simulink model "volo_agcdc_pipelined"  (R2012b)
settings: Solver=ode45  StartTime=0.0  StopTime=1000  RelTol=1e-3
PreLoadFcn:
  | volo_agcdc_init
InitFcn:
  | volo_agcdc_init
StartFcn:
  | volo_agcdc_init
values from neighbouring files (symbols this model uses):
  agc_idleState = 0    [volo_agcdc_init.m]
  agc_numAddrBits = agc_numOutputs + agc_numStateBits    [volo_agcdc_init.m]
  regDCRemoval_AvgLength = 64    [volo_agcdc_init.m]
  regSatDet_NumSamples = 16    [volo_agcdc_init.m]
undefined symbols (not defined in the file or in its folder): gcbh, xlBlockLoadCallback, xlGetNormalizedPeriod
libraries: xbsIndex_r4 x681, xbsEDKLib_r4 x1
(part 1 of 7)
settings Model: Creator=rng  LastModifiedBy=rng

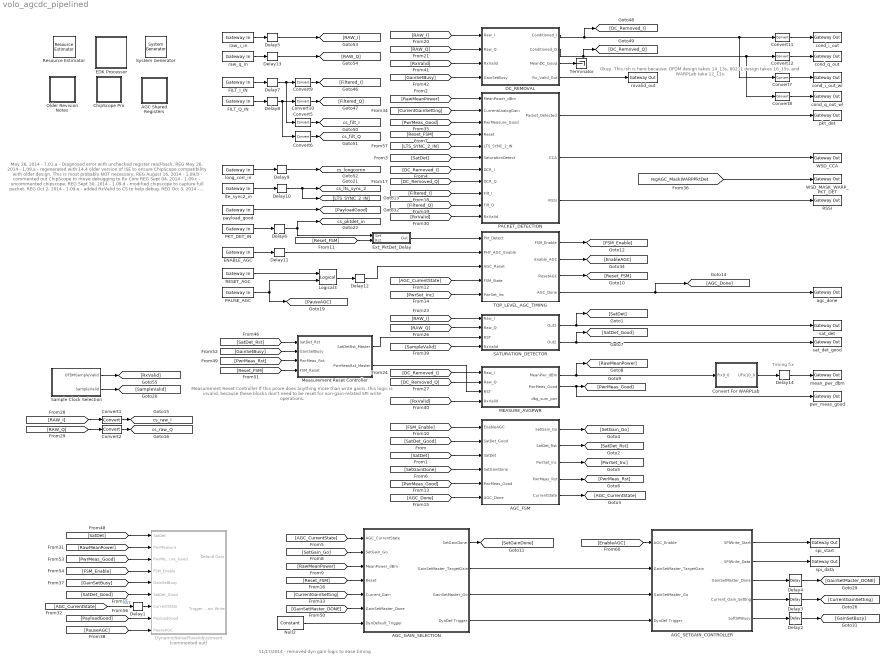
== system volo_agcdc_pipelined ==
  note: 11/17/2014 - removed dyn gain logic to ease timing
  note: Timing fix
  note: Okay. This ish is here because:
      | OFDM design takes 14_13s,
      | 80211 design takes 16_15s,
      | and WARPLab take 12_11s.
  note: May 26, 2014 - 7.01.a - Diagnosed error with unchecked register read-back. REG
      | May 26, 2014 - 1.09.a - regenerated with 14.4 older version of ISE to ensure
      | ChipScope compatibility with older design. This is most probably NOT necessary. REG
      | August 16, 2014 - 1.09.b - commented out ChipScope to move debugging to Rx Core REG
      | Sept 04, 2014 - 1.09.c - uncommented chipscope. REG
      | Sept 30, 2014 - 1.09.d - modified chipscope to capture full packet. REG
      | Oct 2, 2014 - 1.09.e - added RxValid to CS to help debug. REG
      | Oct 3, 2014 - 1.09.f - removed chipscope to wlan_phy_rx. Added RxValid output. REG
      | Nov 16, 2014 - 1.09.g - added a bit of precision to regAGC_WSD_CCAThreshold_dBm
      | MM register to make it Fix_10_0 to match comparison value. Default value now -40 dBm,
      | since the power measurement block does not current consider the external LNA in its input
      | power calculation. In later revisions, we should consider addressing this issue, but for now
      | it is more important that the RSSI and CCA value be relatively accurate and CCA thresh not
      | too low. Also re-enabled chipscope. Added CCA enable line. REG
      | Nov 17, 2014 - 1.09.h - Removed DynDefaultGain functionality to ease timing
      | requirements. REG
      | Jan 01, 2015 - 1.09.j - Added piplining on the SPI go signal, as it was needed when
      | added the 4x1 radio MUX to close timing. REG
  note: Measurement Reset Controller
      | If this pcore does anything more than write gains, this logic is invalid,
      | because these blocks don't need to be reset for non-gain-related SPI
      | write operations.
  " System Generator" : xbsIndex_r4/ System Generator  Tag=genX  xilinxfamily=virtex6  part=xc6vlx240t  speed=-2  package=ff1156  synthesis_tool=XST  clock_wrapper=Clock Enables  directory=./volo_agcdc_generated_pcores  proj_type=Project Navigator  Synth_file=XST Defaults  Impl_file=ISE Defaults  testbench=off  simulink_period=1  sysclk_period=10  dcm_input_clock_period=100  incr_netlist=off  trim_vbits=Everywhere in SubSystem  dbl_ovrd=According to Block Masks  core_generation=According to Block Masks  run_coregen=off  deprecated_control=off  eval_field=0  block_type=sysgen
      settings: block_version=10.1.3
  AGC Shared Registers : Subsystem
  AGC_FSM : Subsystem
  AGC_GAIN_SELECTION : Subsystem
  AGC_SETGAIN_CONTROLLER : Subsystem
  ChipScope Pro : Subsystem
  Convert For WARPLab : Subsystem
  Convert{1..2,5..6} (4 alike) : xbsIndex_r4/Convert  gui_display_data_type=Fixed-point  arith_type="Signed  (2's comp)"  n_bits=12  bin_pt=11  float_type=Single  exp_bits=8  fraction_bits=24  quantization="Round  (unbiased: Even Values)"  overflow=Saturate  en=off  latency=0  dbl_ovrd=off  pipeline=off  block_type=convert
  Convert{7..10} (4 alike) : xbsIndex_r4/Convert  gui_display_data_type=Fixed-point  arith_type="Signed  (2's comp)"  n_bits=12  bin_pt=11  float_type=Single  exp_bits=8  fraction_bits=24  quantization=Truncate  overflow=Wrap  en=off  latency=0  dbl_ovrd=off  pipeline=off  block_type=convert
  Convert11 : xbsIndex_r4/Convert  gui_display_data_type=Fixed-point  arith_type="Signed  (2's comp)"  n_bits=16  bin_pt=15  float_type=Single  exp_bits=8  fraction_bits=24  quantization=Truncate  overflow=Wrap  en=off  latency=0  dbl_ovrd=off  pipeline=off  block_type=convert
  Convert12 : xbsIndex_r4/Convert  gui_display_data_type=Fixed-point  arith_type="Signed  (2's comp)"  n_bits=16  bin_pt=15  float_type=Single  exp_bits=8  fraction_bits=24  quantization=Truncate  overflow=Wrap  en=off  latency=0  dbl_ovrd=off  pipeline=off  block_type=convert
  DC_REMOVAL : Subsystem
  Delay{1,5..14} (11 alike) : xbsIndex_r4/Delay  rst=off  infoeditControl=Selection of Reset will increase slice count due to use of real FFs and instead of SRLs  en=off  latency=1  dbl_ovrd=off  reg_retiming=off  block_type=delay
  Delay2 : xbsIndex_r4/Delay  rst=off  infoeditControl=Selection of Reset will increase slice count due to use of real FFs and instead of SRLs  en=off  latency=2  dbl_ovrd=off  reg_retiming=off  block_type=delay
  Delay3 : xbsIndex_r4/Delay  rst=off  infoeditControl=Selection of Reset will increase slice count due to use of real FFs and instead of SRLs  en=off  latency=2  dbl_ovrd=off  reg_retiming=off  block_type=delay
  Delay4 : xbsIndex_r4/Delay  rst=off  infoeditControl=Selection of Reset will increase slice count due to use of real FFs and instead of SRLs  en=off  latency=2  dbl_ovrd=off  reg_retiming=off  block_type=delay
  DynamicNoiseFloorAdjustment : Subsystem  Commented=on
  EDK Processor : Subsystem  LoadFcn=xlBlockLoadCallback(gcbh);  mask(Xilinx EDK Processor Block){mode=EDK pcore generation, xmp=, MemVisToProc=<qt bgcolor="#FFFFFF"><div><img src="E:/Xilinx_ISE_14_4/14.4/ISE_DS/ISE/sysgen/data/images/registerplus.gif"> &lt;&lt;regAGC_DefaultGainSettings&gt;&gt;<br></div><div><img src="E:/Xilinx_ISE_14_4/14.4/ISE_DS/ISE/sysgen/data/images/registerplus.gif"> &lt;&lt;regSPICtrl_SPIWriteDelay&gt;&gt;<br></div><div><img src="E:/Xilinx_ISE_14_4/14.4/ISE_DS/ISE/sysgen/data/images/registerplus.gif"> &lt;&lt;regPwrMeas_AvgLength&gt;&gt;<br></div><div><img src="E:/Xilinx_ISE_14_4/14.4/ISE_DS/ISE/sysgen/data/images/registerplus.gif"> &lt;&lt;regSatDet_SaturationMaxCount&gt;&gt;<br></div><div><img src="E:/Xilinx_ISE_14_4/14.4/ISE_DS/ISE/sysgen/data/images/registerplus.gif"> &lt;&lt;regSatDet_NumSamples&gt;&gt;<br></div><div><img src="E:/Xilinx_ISE_14_4/14.4/ISE_DS/ISE/sysgen/data/images/registerplus.gif"> &lt;&lt;regSatDet_SaturationThreshold&gt;&gt;<br></div><div><img src="E:/Xilinx_ISE_14_4/14.4/ISE_DS/ISE/sysgen/data/images/registerplus.gif"> &lt;&lt;regAGC_ExtPktDet_DelayCount&gt;&gt;<br></div><div><img src="E:/Xilinx_ISE_14_4/14.4/ISE_DS/ISE/sysgen/data/images/registerplus.gif"> &lt;&lt;regAGC_targetRxInputPwr&gt;&gt;<br></div><div><img src="E:/Xilinx_ISE_14_4/14.4/ISE_DS/ISE/sysgen/data/images/registerplus.gif"> &lt;&lt;regAGC_AutoCorr_MinPower&gt;&gt;<br></div><div><img src="E:/Xilinx_ISE_14_4/14.4/ISE_DS/ISE/sysgen/data/images/registerplus.gif"> &lt;&lt;regAGC_AutoCorr_MinPktDuration&gt;&gt;<br></div><div><img src="E:/Xilinx_ISE_14_4/14.4/ISE_DS/ISE/sysgen/data/images/registerplus.gif"> &lt;&lt;regAGC_WSDAGCCtrl&gt;&gt;<br></div><div><img src="E:/Xilinx_ISE_14_4/14.4/ISE_DS/ISE/sysgen/data/images/registerplus.gif"> &lt;&lt;regAGC_AutoCorr_RatioThresh&gt;&gt;<br></div><div><img src="E:/Xilinx_ISE_14_4/14.4/ISE_DS/ISE/sysgen/data/images/registerplus.gif"> &lt;&lt;regAGC_ManualRxVGA1_Gain&gt;&gt;<br></div><div><img src="E:/Xilinx_ISE_14_4/14.4/ISE_DS/ISE/sysgen/data/images/registerplus.gif"> &lt;&lt;regAGC_ManualRxLNA_Gain&gt;&gt;<br></div><div><img src="E:/Xilinx_ISE_14_4/14.4/ISE_DS/ISE/sysgen/data/images/registerplus.gif"> &lt;&lt;regAGC_ManualRxVGA2_Gain&gt;&gt;<br></div><div><img src="E:/Xilinx_ISE_14_4/14.4/ISE_DS/ISE/sysgen/data/images/registerplus.gif"> &lt;&lt;regAGC_AutoCorr_LagTime&gt;&gt;<br></div><div><img src="E:/Xilinx_ISE_14_4/14.4/ISE_DS/ISE/sysgen/data/images/registerplus.gif"> &lt;&lt;regAGC_pktDetPwr_absoluteThreshold_dBm&gt;&gt;<br></div><div><img src="E:/Xilinx_ISE_14_4/14.4/ISE_DS/ISE/sysgen/data/images/registerplus.gif"> &lt;&lt;regAGC_pktDetPwr_detectLag&gt;&gt;<br></div><div><img src="E:/Xilinx_ISE_14_4/14.4/ISE_DS/ISE/sysgen/data/images/registerplus.gif"> &lt;&lt;regAGC_NumFineGainSteps&gt;&gt;<br></div><div><img src="E:/Xilinx_ISE_14_4/14.4/ISE_DS/ISE/sysgen/data/images/registerplus.gif"> &lt;&lt;regAGC_WSD_CCAThreshold_dBm&gt;&gt;<br></div><div><img src="E:/Xilinx_ISE_14_4/14.4/ISE_DS/ISE/sysgen/data/images/registerplus.gif"> &lt;&lt;regAGC_LongCorr_Threshold&gt;&gt;<br></div><div><img src="E:/Xilinx_ISE_14_4/14.4/ISE_DS/ISE/sysgen/data/images/registerplus.gif"> &lt;&lt;regAGC_pktDetPwr_deltaThreshold_dBm&gt;&gt;<br></div><div><img src="E:/Xilinx_ISE_14_4/14.4/ISE_DS/ISE/sysgen/data/images/registerplus.gif"> &lt;&lt;regAGC_SPITIMINGFUDGE&gt;&gt;<br></div><div><img src="E:/Xilinx_ISE_14_4/14.4/ISE_DS/ISE/sysgen/data/images/registerplus.gif"> &lt;&lt;regSatDet_SaturationDetected&gt;&gt;<br></div><div><img src="E:/Xilinx_ISE_14_4/14.4/ISE_DS/ISE/sysgen/data/images/registerplus.gif"> &lt;&lt;regWSD_RXGAIN_READ&gt;&gt;<br></div><div><img src="E:/Xilinx_ISE_14_4/14.4/ISE_DS/ISE/sysgen/data/images/registerplus.gif"> &lt;&lt;regWSD_RSSI&gt;&gt;<br></div><div><img src="E:/Xilinx_ISE_14_4/14.4/ISE_DS/ISE/sysgen/data/images/registerplus.gif"> &lt;&lt;regWSD_meanPower&gt;&gt;<br></div><div><img src="E:/Xilinx_ISE_14_4/14.4/ISE_DS/ISE/sysgen/data/images/registerplus.gif"> &lt;&lt;regWSD_MeanDC_Q&gt;&gt;<br></div><div><img src="E:/Xilinx_ISE_14_4/14.4/ISE_DS/ISE/sysgen/data/images/registerplus.gif"> &lt;&lt;regWSD_MeanDC_I&gt;&gt;<br></div><div><img src="E:/Xilinx_ISE_14_4/14.4/ISE_DS/ISE/sysgen/data/images/registerplus.gif"> &lt;&lt;regWSD_RxLNAGain&gt;&gt;<br></div><div><img src="E:/Xilinx_ISE_14_4/14.4/ISE_DS/ISE/sysgen/data/images/registerplus.gif"> &lt;&lt;regWSD_RxVGA1Gain&gt;&gt;<br></div><div><img src="E:/Xilinx_ISE_14_4/14.4/ISE_DS/ISE/sysgen/data/images/registerplus.gif"> &lt;&lt;regWSD_RxVGA2Gain&gt;&gt;<br></div></qt>, AvailableMemories=<empty>, portInterfaceTable={'exposed'=>[],'portdir'=>[],'portname'=>[],'shortname'=>[]}, bus_type_sgadvanced=, bus_type=AXI, baseaddr=0x80000000, baseaddr_lock_sgadvanced=, baseaddr_lock=off, dual_clock_sgadvanced=, dual_clock=on, reg_readback_sgadvanced=, reg_readback=on, ucf_file=, inheritDeviceType_sgadvanced=, inheritDeviceType=off, elf_file=, codebug_sgadvanced=, codebug=on, clock_name=plb, internalPortList={}, resetPolarity=0, memxtable={'mladdr'=>[0.00000000000000000,1.00000000000000000,2.00000000000000000,3.00000000000000000,4.00000000000000000,5.00000000000000000,6.00000000000000000,7.00000000000000000,8.00000000000000000,9.00000000000000000,10.00000000000000000,11.00000000000000000,12.00000000000000000,13.00000000000000000,14.00000000000000000,15.00000000000000000,16.00000000000000000,17.00000000000000000,18.00000000000000000,19.00000000000000000,20.00000000000000000,21.00000000000000000,22.00000000000000000,0.00000000000000000,1.00000000000000000,2.00000000000000000,3.00000000000000000,4.00000000000000000,5.00000000000000000,6.00000000000000000,7.00000000000000000,8.00000000000000000],'mlist'=>['volo_agcdc_pipelined/AGC Shared Registers/From Register9','volo_agcdc_pipelined/AGC Shared Registers/From Register8','volo_agcdc_pipelined/AGC Shared Registers/From Register7','volo_agcdc_pipelined/AGC Shared Registers/From Register6','volo_agcdc_pipelined/AGC Shared Registers/From Register5','volo_agcdc_pipelined/AGC Shared Registers/From Register4','volo_agcdc_pipelined/AGC Shared Registers/From Register30','volo_agcdc_pipelined/AGC Shared Registers/From Register3','volo_agcdc_pipelined/AGC Shared Registers/From Register28','volo_agcdc_pipelined/AGC Shared Registers/From Register27','volo_agcdc_pipelined/AGC Shared Registers/From Register26','volo_agcdc_pipelined/AGC Shared Registers/From Register25','volo_agcdc_pipelined/AGC Shared Registers/From Register24','volo_agcdc_pipelined/AGC Shared Registers/From Register23','volo_agcdc_pipelined/AGC Shared Registers/From Register22','volo_agcdc_pipelined/AGC Shared Registers/From Register2','volo_agcdc_pipelined/AGC Shared Registers/From Register17','volo_agcdc_pipelined/AGC Shared Registers/From Register16','volo_agcdc_pipelined/AGC Shared Registers/From Register14','volo_agcdc_pipelined/AGC Shared Registers/From Register12','volo_agcdc_pipelined/AGC Shared Registers/From Register11','volo_agcdc_pipelined/AGC Shared Registers/From Register10','volo_agcdc_pipelined/AGC Shared Registers/From Register','volo_agcdc_pipelined/SATURATION_DETECTOR/To Register','volo_agcdc_pipelined/PACKET_DETECTION/To Register1','volo_agcdc_pipelined/PACKET_DETECTION/To Register','volo_agcdc_pipelined/MEASURE_AVGPWR/To Register','volo_agcdc_pipelined/DC_REMOVAL/To Register1','volo_agcdc_pipelined/DC_REMOVAL/To Register','volo_agcdc_pipelined/AGC_SETGAIN_CONTROLLER/To Register2','volo_agcdc_pipelined/AGC_SETGAIN_CONTROLLER/To Register1','volo_agcdc_pipelined/AGC_SETGAIN_CONTROLLER/To Register'],'mlname'=>['\'regAGC_DefaultGainSettings\'','\'regSPICtrl_SPIWriteDelay\'','\'regPwrMeas_AvgLength\'','\'regSatDet_SaturationMaxCount\'','\'regSatDet_NumSamples\'','\'regSatDet_SaturationThreshold\'','\'regAGC_ExtPktDet_DelayCount\'','\'regAGC_targetRxInputPwr\'','\'regAGC_AutoCorr_MinPower\'','\'regAGC_AutoCorr_MinPktDuration\'','\'regAGC_WSDAGCCtrl\'','\'regAGC_AutoCorr_RatioThresh\'','\'regAGC_ManualRxVGA1_Gain\'','\'regAGC_ManualRxLNA_Gain\'','\'regAGC_ManualRxVGA2_Gain\'','\'regAGC_AutoCorr_LagTime\'','\'regAGC_pktDetPwr_absoluteThreshold_dBm\'','\'regAGC_pktDetPwr_detectLag\'','\'regAGC_NumFineGainSteps\'','\'regAGC_WSD_CCAThreshold_dBm\'','\'regAGC_LongCorr_Threshold\'','\'regAGC_pktDetPwr_deltaThreshold_dBm\'','\'regAGC_SPITIMINGFUDGE\'','\'regSatDet_SaturationDetected\'','\'regWSD_RXGAIN_READ\'','\'regWSD_RSSI\'','\'regWSD_meanPower\'','\'regWSD_MeanDC_Q\'','\'regWSD_MeanDC_I\'','\'regWSD_RxLNAGain\'','\'regWSD_RxVGA1Gain\'','\'regWSD_RxVGA2Gain\''],'mlstate'=>[0.00000000000000000,0.00000000000000000,0.00000000000000000,0.00000000000000000,0.00000000000000000,0.00000000000000000,0.00000000000000000,0.00000000000000000,0.00000000000000000,0.00000000000000000,0.00000000000000000,0.00000000000000000,0.00000000000000000,0.00000000000000000,0.00000000000000000,0.00000000000000000,0.00000000000000000,0.00000000000000000,0.00000000000000000,0.00000000000000000,0.00000000000000000,0.00000000000000000,0.00000000000000000,0.00000000000000000,0.00000000000000000,0.00000000000000000,0.00000000000000000,0.00000000000000000,0.00000000000000000,0.00000000000000000,0.00000000000000000,0.00000000000000000]}, procinfo={}, memmapdirty=off, blockname=, xpsintstyle=default, has_advanced_control=0, sggui_pos=-1928,-8,1920,1058, block_type=edkprocessor, block_version=2.7, sg_icon_stat=62,64,-1,-1,white,blue,0,07734,right,,[ ],[ ], sg_mask_display=|, sg_list_contents={'table'=>{'AvailableMemories'=>'popup(<empty>)'}}, sg_blockgui_xml=}
      mask sg_mask_display=|
      | fprintf('','COMMENT: begin icon graphics');
      | patch([0 62 62 0 0 ],[0 0 64 64 0 ],[0.77 0.82 0.91 ]);
      | plot([0 62 62 0 0 ],[0 0 64 64 0 ]);
      | patch([13.2 24.76 32.76 40.76 48.76 32.76 21.2 13.2 ],[40.88 40.88 48.88 40.88 48.88 48.88 48.88 40.88 ],[1 1 1 ]);
      | patch([21.2 32.76 24.76 13.2 21.2 ],[32.88 32.88 40.88 40.88 32.88 ],[0.931 0.946 0.973 ]);
      | patch([13.2 24.76 32.76 21.2 13.2 ],[24.88 24.88 32.88 32.88 24.88 ],[1 1 1 ]);
      | patch([21.2 48.76 40.76 32.76 24.76 13.2 21.2 ],[16.88 16.88 24.88 16.88 24.88 24.88 16.88 ],[0.931 0.946 0.973 ]);
      | fprintf('','COMMENT: end icon graphics');
      | fprintf('','COMMENT: begin icon text');
      | fprintf('','COMMENT: end icon text');
      mask prompts: mode "Configure Processor for"; xmp "XPS Project"; MemVisToProc ""; AvailableMemories "Available Memories"; portInterfaceTable ""; bus_type_sgadvanced ""; bus_type "Bus Type"; baseaddr "Base Address"; baseaddr_lock_sgadvanced ""; baseaddr_lock "Lock"; dual_clock_sgadvanced ""; dual_clock "Dual Clocks"; reg_readback_sgadvanced ""; reg_readback "Register Read-Back"; ucf_file "Constraint File"; inheritDeviceType_sgadvanced ""; inheritDeviceType "Inherit Device Type"; elf_file "Initial Program"; codebug_sgadvanced ""; codebug "Enable Co-Debug with Xilinx SDK (Beta)"; clock_name ""; internalPortList ""; resetPolarity ""; memxtable ""; procinfo ""; memmapdirty ""; blockname ""; xpsintstyle ""; has_advanced_control ""; sggui_pos ""; block_type ""; block_version ""; sg_icon_stat ""; sg_mask_display ""; sg_list_contents ""; sg_blockgui_xml ""
      mask help: Xilinx EDK Processor
      mask init:
      | try
      |   tmp_gcb = gcb;
      |   tmp_gcbh = gcbh;
      |   if (strcmp('SysGenIndex',get_param(bdroot(tmp_gcbh),'tag')) && ~isempty(regexp(bdroot(tmp_gcb), '^xbs', 'once')))
      |     return;
      |   end;
      |   xlMungeMaskParams;
      | 
      |   block_type='edkprocessor';
      | 
      |   serialized_declarations = '{''block_type''=>''String''}';
      |   xledkprocessor_init();
      |   ptable_ = xlblockprep(get_param(tmp_gcb, 'MaskWSVariables'));
      |   try
      |     xlBlockMoveCallback(tmp_gcbh);
      |   catch 
      |      clear global xl_updateicon_recursion_guard;
      |   end;
      | catch
      |   global dbgsysgen;
      |   if(~isempty(dbgsysgen) && dbgsysgen)
      |     e = regexprep(lasterr, '\n', '\nError: ');
      |     disp(['Error: While running MaskInit code on block ' tmp_gcb ': ' e]);
      |     error(e);
      |   end
      | end
      settings: CopyFcn=xlProcBlockCopyCallback(gcbh);xlBlockMoveCallback(gcbh);  DeleteFcn=xlDestroyGui(gcbh);  ModelCloseFcn=xlDestroyGui(gcbh);  PreSaveFcn=xlBlockPreSaveCallback(gcbh);  PostSaveFcn=xlBlockPostSaveCallback(gcbh);  DestroyFcn=xlDestroyGui(gcbh);  OpenFcn=bh=gcbh;xlProcBlockCallbacks('populatesharedmemorylistbox',bh);xlOpenGui(bh, 'edkprocessor_gui.xml', @xlProcBlockEnablement, @xlProcBlockAction);  CloseFcn=xlDestroyGui(gcbh);  MoveFcn=xlBlockMoveCallback(gcbh);
      mask Help: eval('');xlDoc('-book','sysgen','-topic','EDK_Processor');
      mask TypeOptions mode: EDK pcore generation | HDL netlisting
      mask TypeOptions bus_type: AXI | PLB
      mask Display:
      | fprintf('','COMMENT: begin icon graphics');
      | patch([0 62 62 0 0 ],[0 0 64 64 0 ],[0.77 0.82 0.91 ]);
      | plot([0 62 62 0 0 ],[0 0 64 64 0 ]);
      | patch([13.2 24.76 32.76 40.76 48.76 32.76 21.2 13.2 ],[40.88 40.88 48.88 40.88 48.88 48.88 48.88 40.88 ],[1 1 1 ]);
      | patch([21.2 32.76 24.76 13.2 21.2 ],[32.88 32.88 40.88 40.88 32.88 ],[0.931 0.946 0.973 ]);
      | patch([13.2 24.76 32.76 21.2 13.2 ],[24.88 24.88 32.88 32.88 24.88 ],[1 1 1 ]);
      | patch([21.2 48.76 40.76 32.76 24.76 13.2 21.2 ],[16.88 16.88 24.88 16.88 24.88 24.88 16.88 ],[0.931 0.946 0.973 ]);
      | fprintf('','COMMENT: end icon graphics');
      | fprintf('','COMMENT: begin icon text');
      | disp('');
      | 
      | fprintf('','COMMENT: end icon text');
  ENABLE_AGC : xbsIndex_r4/Gateway In  gui_display_data_type=Boolean  arith_type=Boolean  n_bits=14  bin_pt=13  preci_type=Single  exp_width=8  frac_width=24  quantization="Round  (unbiased: +/- Inf)"  overflow=Saturate  period=1  dbl_ovrd=off  timing_constraint=None  locs_specified=off  LOCs={}  UseAsADC=off  ADCChannel='1'  inherit_from_input=off  hdl_port=on  block_type=gatewayin
  Ext_PktDet_Delay : Subsystem
  FILT_I_IN : xbsIndex_r4/Gateway In  gui_display_data_type=Fixed-point  arith_type="Signed  (2's comp)"  n_bits=16  bin_pt=15  preci_type=Single  exp_width=8  frac_width=24  quantization="Round  (unbiased: +/- Inf)"  overflow=Saturate  period=1  dbl_ovrd=off  timing_constraint=None  locs_specified=off  LOCs={}  UseAsADC=off  ADCChannel='1'  inherit_from_input=off  hdl_port=on  block_type=gatewayin
  FILT_Q_IN : xbsIndex_r4/Gateway In  gui_display_data_type=Fixed-point  arith_type="Signed  (2's comp)"  n_bits=16  bin_pt=15  preci_type=Single  exp_width=8  frac_width=24  quantization="Round  (unbiased: +/- Inf)"  overflow=Saturate  period=1  dbl_ovrd=off  timing_constraint=None  locs_specified=off  LOCs={}  UseAsADC=off  ADCChannel='1'  inherit_from_input=off  hdl_port=on  block_type=gatewayin
  Logical3 : xbsIndex_r4/Logical  logical_function=OR  inputs=2  en=off  latency=0  precision=Full  arith_type=Unsigned  n_bits=16  bin_pt=0  align_bp=on  dbl_ovrd=off  block_type=logical
  MEASURE_AVGPWR : Subsystem
  Measurement Reset Controller : Subsystem
  Null2 : xbsIndex_r4/Constant  const=0  gui_display_data_type=Boolean  arith_type=Boolean  n_bits=3  bin_pt=0  preci_type=Single  exp_width=8  frac_width=24  explicit_period=off  period=1  equ=P=C  opselect=C  inp2=PCIN>>17  opr=+  inp1=P  carry=CIN  dbl_ovrd=off  block_type=constant
  Older Revision Notes : Subsystem
  PACKET_DETECTION : Subsystem
  PAUSE_AGC : xbsIndex_r4/Gateway In  gui_display_data_type=Boolean  arith_type=Boolean  n_bits=14  bin_pt=13  preci_type=Single  exp_width=8  frac_width=24  quantization="Round  (unbiased: +/- Inf)"  overflow=Saturate  period=1  dbl_ovrd=off  timing_constraint=None  locs_specified=off  LOCs={}  UseAsADC=off  ADCChannel='1'  inherit_from_input=off  hdl_port=on  block_type=gatewayin
  PKT_DET_IN : xbsIndex_r4/Gateway In  gui_display_data_type=Boolean  arith_type=Boolean  n_bits=14  bin_pt=13  preci_type=Single  exp_width=8  frac_width=24  quantization="Round  (unbiased: +/- Inf)"  overflow=Saturate  period=1  dbl_ovrd=off  timing_constraint=None  locs_specified=off  LOCs={}  UseAsADC=off  ADCChannel='1'  inherit_from_input=off  hdl_port=on  block_type=gatewayin
  RESET_AGC : xbsIndex_r4/Gateway In  gui_display_data_type=Boolean  arith_type=Boolean  n_bits=14  bin_pt=13  preci_type=Single  exp_width=8  frac_width=24  quantization="Round  (unbiased: +/- Inf)"  overflow=Saturate  period=1  dbl_ovrd=off  timing_constraint=None  locs_specified=off  LOCs={}  UseAsADC=off  ADCChannel='1'  inherit_from_input=off  hdl_port=on  block_type=gatewayin
  RSSI : xbsIndex_r4/Gateway Out  inherit_from_input=off  hdl_port=on  timing_constraint=None  locs_specified=off  LOCs={}  UseAsDAC=off  DACChannel='1'  block_type=gatewayout
  Resource Estimator : xbsIndex_r4/Resource Estimator  Tag=resEstTag  Slices=3628  FFs=4465  BRAMs=0  LUTs=6136  IOBs=365  EBMs=48  TBUFs=0  xl_use_estimator_area=off  est_options=Post Map  xl_estimator_area=[3628 4465 0 6136 365 48 0]  block_type=resource_estimator
      settings: AttributesFormatString=Resource\nEstimator  block_version=10.1.3
  SATURATION_DETECTOR : Subsystem
  Sample Clock Selection : Subsystem
  TOP_LEVEL_AGC_TIMING : Subsystem
  Terminator : Terminator
  WSD_CCA : xbsIndex_r4/Gateway Out  inherit_from_input=on  hdl_port=on  timing_constraint=None  locs_specified=off  LOCs={}  UseAsDAC=off  DACChannel='1'  block_type=gatewayout
  WSD_MASK_WARP_PKT_DET : xbsIndex_r4/Gateway Out  inherit_from_input=off  hdl_port=on  timing_constraint=None  locs_specified=off  LOCs={}  UseAsDAC=off  DACChannel='1'  block_type=gatewayout
  agc_done : xbsIndex_r4/Gateway Out  inherit_from_input=off  hdl_port=on  timing_constraint=None  locs_specified=off  LOCs={}  UseAsDAC=off  DACChannel='1'  block_type=gatewayout
  cond_i_out : xbsIndex_r4/Gateway Out  inherit_from_input=off  hdl_port=on  timing_constraint=None  locs_specified=off  LOCs={}  UseAsDAC=off  DACChannel='1'  block_type=gatewayout
  cond_i_out_wl : xbsIndex_r4/Gateway Out  inherit_from_input=off  hdl_port=on  timing_constraint=None  locs_specified=off  LOCs={}  UseAsDAC=off  DACChannel='1'  block_type=gatewayout
  cond_q_out : xbsIndex_r4/Gateway Out  inherit_from_input=off  hdl_port=on  timing_constraint=None  locs_specified=off  LOCs={}  UseAsDAC=off  DACChannel='1'  block_type=gatewayout
  cond_q_out_wl : xbsIndex_r4/Gateway Out  inherit_from_input=off  hdl_port=on  timing_constraint=None  locs_specified=off  LOCs={}  UseAsDAC=off  DACChannel='1'  block_type=gatewayout
  long_corr_in : xbsIndex_r4/Gateway In  gui_display_data_type=Fixed-point  arith_type=Unsigned  n_bits=32  bin_pt=0  preci_type=Single  exp_width=8  frac_width=24  quantization="Round  (unbiased: +/- Inf)"  overflow=Saturate  period=1  dbl_ovrd=off  timing_constraint=None  locs_specified=off  LOCs={}  UseAsADC=off  ADCChannel='1'  inherit_from_input=off  hdl_port=on  block_type=gatewayin
  lte_sync2_in : xbsIndex_r4/Gateway In  gui_display_data_type=Boolean  arith_type=Boolean  n_bits=32  bin_pt=0  preci_type=Single  exp_width=8  frac_width=24  quantization="Round  (unbiased: +/- Inf)"  overflow=Saturate  period=1  dbl_ovrd=off  timing_constraint=None  locs_specified=off  LOCs={}  UseAsADC=off  ADCChannel='1'  inherit_from_input=off  hdl_port=on  block_type=gatewayin
  mean_pwr_dbm : xbsIndex_r4/Gateway Out  inherit_from_input=off  hdl_port=on  timing_constraint=None  locs_specified=off  LOCs={}  UseAsDAC=off  DACChannel='1'  block_type=gatewayout
  payload_good : xbsIndex_r4/Gateway In  gui_display_data_type=Boolean  arith_type=Boolean  n_bits=14  bin_pt=13  preci_type=Single  exp_width=8  frac_width=24  quantization="Round  (unbiased: +/- Inf)"  overflow=Saturate  period=1  dbl_ovrd=off  timing_constraint=None  locs_specified=off  LOCs={}  UseAsADC=off  ADCChannel='1'  inherit_from_input=off  hdl_port=on  block_type=gatewayin
  pkt_det : xbsIndex_r4/Gateway Out  inherit_from_input=off  hdl_port=on  timing_constraint=None  locs_specified=off  LOCs={}  UseAsDAC=off  DACChannel='1'  block_type=gatewayout
  pwr_meas_good : xbsIndex_r4/Gateway Out  inherit_from_input=on  hdl_port=on  timing_constraint=None  locs_specified=off  LOCs={}  UseAsDAC=off  DACChannel='1'  block_type=gatewayout
  raw_i_in : xbsIndex_r4/Gateway In  gui_display_data_type=Fixed-point  arith_type="Signed  (2's comp)"  n_bits=12  bin_pt=11  preci_type=Single  exp_width=8  frac_width=24  quantization="Round  (unbiased: +/- Inf)"  overflow=Saturate  period=1  dbl_ovrd=off  timing_constraint=None  locs_specified=off  LOCs={}  UseAsADC=off  ADCChannel='1'  inherit_from_input=off  hdl_port=on  block_type=gatewayin
  raw_q_in : xbsIndex_r4/Gateway In  gui_display_data_type=Fixed-point  arith_type="Signed  (2's comp)"  n_bits=12  bin_pt=11  preci_type=Single  exp_width=8  frac_width=24  quantization="Round  (unbiased: +/- Inf)"  overflow=Saturate  period=1  dbl_ovrd=off  timing_constraint=None  locs_specified=off  LOCs={}  UseAsADC=off  ADCChannel='1'  inherit_from_input=off  hdl_port=on  block_type=gatewayin
  rxvalid_out : xbsIndex_r4/Gateway Out  inherit_from_input=off  hdl_port=on  timing_constraint=None  locs_specified=off  LOCs={}  UseAsDAC=off  DACChannel='1'  block_type=gatewayout
  sat_det : xbsIndex_r4/Gateway Out  inherit_from_input=off  hdl_port=on  timing_constraint=None  locs_specified=off  LOCs={}  UseAsDAC=off  DACChannel='1'  block_type=gatewayout
  sat_det_good : xbsIndex_r4/Gateway Out  inherit_from_input=off  hdl_port=off  timing_constraint=None  locs_specified=off  LOCs={}  UseAsDAC=off  DACChannel='1'  block_type=gatewayout
  spi_data : xbsIndex_r4/Gateway Out  inherit_from_input=off  hdl_port=on  timing_constraint=None  locs_specified=off  LOCs={}  UseAsDAC=off  DACChannel='1'  block_type=gatewayout
  spi_start : xbsIndex_r4/Gateway Out  inherit_from_input=off  hdl_port=on  timing_constraint=None  locs_specified=off  LOCs={}  UseAsDAC=off  DACChannel='1'  block_type=gatewayout
  tag scope: cs_filt_I=global, cs_filt_Q=global, cs_longcorrin=global, cs_lts_sync_2=global, cs_pktdet_in=global, cs_raw_I=global, cs_raw_Q=global
  wires:
  SATURATION_DETECTOR/1(Out1) -> [SatDet], sat_det/1
  AGC_FSM/5(CurrentState) -> [AGC_CurrentState]
  AGC_FSM/1(SetGain_Go) -> [SetGain_Go]
  AGC_FSM/2(SatDet_Rst) -> [SatDet_Rst]
  AGC_FSM/3(PwrSet_Inc) -> [PwrSet_Inc]
  AGC_FSM/4(PwrMeas_Rst) -> [PwrMeas_Rst]
  [SatDet_Good] -> AGC_FSM/2(SatDet_Good)
  [SatDet] -> AGC_FSM/3(SatDet)
  [SetGainDone] -> AGC_FSM/4(SetGainDone)
  [PwrMeas_Good] -> AGC_FSM/5(PwrMeas_Good)
  MEASURE_AVGPWR/2(PwrMeas_Good) -> pwr_meas_good/1, [PwrMeas_Good]
  SATURATION_DETECTOR/2(Out2) -> [SatDet_Good], sat_det_good/1
  AGC_GAIN_SELECTION/1(SetGainDone) -> [SetGainDone]
  [RawMeanPower] -> AGC_GAIN_SELECTION/3(MeanPower_dBm)
  [AGC_CurrentState] -> AGC_GAIN_SELECTION/1(AGC_CurrentState)
  [SetGain_Go] -> AGC_GAIN_SELECTION/2(SetGain_Go)
  AGC_GAIN_SELECTION/2(GainSetMaster_TargetGain) -> AGC_SETGAIN_CONTROLLER/2(GainSetMaster_TargetGain)
  AGC_SETGAIN_CONTROLLER/1(SPIWrite_Start) -> spi_start/1
  AGC_SETGAIN_CONTROLLER/2(SPIWrite_Data) -> spi_data/1
  DC_REMOVAL/1(Conditioned_I) -> Convert7/1, Convert11/1, [DC_Removed_I]
  DC_REMOVAL/2(Conditioned_Q) -> Convert8/1, Convert12/1, [DC_Removed_Q]
  PACKET_DETECTION/1(Packet_Detected) -> pkt_det/1
  [FSM_Enable] -> AGC_FSM/1(EnableAGC)
  DC_REMOVAL/3(MeanDC_Good) -> Terminator/1
  [AGC_Done] -> AGC_FSM/6(AGC_Done)
  [Reset_FSM] -> AGC_GAIN_SELECTION/4(Reset)
  MEASURE_AVGPWR/1(MeanPwr_dBm) -> Convert For WARPLab/1(Fix9_0), [RawMeanPower]
  Convert1/1 -> [cs_raw_I]
  Convert2/1 -> [cs_raw_Q]
  AGC_SETGAIN_CONTROLLER/4(Current_Gain_Setting) -> Delay3/1
  [RawMeanPower] -> PACKET_DETECTION/1(MeanPower_dBm)
  [Reset_FSM] -> PACKET_DETECTION/4(Reset)
  [CurrentGainSetting] -> PACKET_DETECTION/2(CurrentAnalogGain)
  [PwrMeas_Good] -> PACKET_DETECTION/3(PwrMeasure_Good)
  [CurrentGainSetting] -> AGC_GAIN_SELECTION/5(Current_Gain)
  [GainSetBusy] -> Measurement Reset Controller/2(GainSetBusy)
  Measurement Reset Controller/1(SatDetRst_Master) -> SATURATION_DETECTOR/3(RST)
  Measurement Reset Controller/2(PwrMeasRst_Master) -> MEASURE_AVGPWR/3(RST)
  [PwrMeas_Rst] -> Measurement Reset Controller/3(PwrMeas_Rst)
  [SatDet_Rst] -> Measurement Reset Controller/1(SatDet_Rst)
  AGC_SETGAIN_CONTROLLER/5(SoftSPIBusy) -> Delay2/1
  AGC_SETGAIN_CONTROLLER/3(GainSetMaster_Done) -> Delay4/1
  [GainSetMaster_DONE] -> AGC_GAIN_SELECTION/6(GainSetMaster_Done)
  [Reset_FSM] -> Measurement Reset Controller/4(FSM_Reset)
  payload_good/1 -> [PayloadGood]
  [LTS_SYNC_2_IN] -> PACKET_DETECTION/5(LTS_SYNC_2_IN)
  PACKET_DETECTION/3(RSSI) -> RSSI/1
  [EnableAGC] -> AGC_SETGAIN_CONTROLLER/1(AGC_Enable)
  [SatDet] -> PACKET_DETECTION/6(SaturationDetect)
  FILT_I_IN/1 -> Delay7/1
  FILT_Q_IN/1 -> Delay8/1
  [DC_Removed_I] -> PACKET_DETECTION/7(DCR_I)
  [DC_Removed_Q] -> PACKET_DETECTION/8(DCR_Q)
  [Filtered_I] -> PACKET_DETECTION/9(Filt_I)
  [Filtered_Q] -> PACKET_DETECTION/10(Filt_Q)
  Convert5/1 -> [cs_filt_I]
  Convert6/1 -> [cs_filt_Q]
  [RAW_I] -> DC_REMOVAL/1(Raw_I)
  [RAW_Q] -> DC_REMOVAL/2(Raw_Q)
  Convert9/1 -> [Filtered_I]
  Convert10/1 -> [Filtered_Q]
  Convert11/1 -> cond_i_out/1
  Convert12/1 -> cond_q_out/1
  [RAW_I] -> SATURATION_DETECTOR/1(Raw_I)
  [DC_Removed_I] -> MEASURE_AVGPWR/1(Raw_I)
  [RAW_Q] -> SATURATION_DETECTOR/2(Raw_Q)
  [DC_Removed_Q] -> MEASURE_AVGPWR/2(Raw_Q)
  [RAW_I] -> Convert1/1
  [RAW_Q] -> Convert2/1
  Sample Clock Selection/1(OFDMSampleValid) -> [RxValid]
  [RxValid] -> PACKET_DETECTION/11(RxValid)
  [AGC_CurrentState] -> Delay1/1  "RST"
  [PwrMeas_Good] -> DynamicNoiseFloorAdjustment/3(PwrMeasure_Good)
  [SatDet_Good] -> DynamicNoiseFloorAdjustment/6(SatDet_Good)
  [PayloadGood] -> DynamicNoiseFloorAdjustment/8(PayloadGood)
  [SatDet] -> DynamicNoiseFloorAdjustment/1(SatDet)
  [RawMeanPower] -> DynamicNoiseFloorAdjustment/2(PwrMeasure)
  [FSM_Enable] -> DynamicNoiseFloorAdjustment/4(FSM_Enable)
  AGC_GAIN_SELECTION/3(GainSetMaster_Go) -> AGC_SETGAIN_CONTROLLER/3(GainSetMaster_Go)
  AGC_GAIN_SELECTION/4(DynDef Trigger) -> AGC_SETGAIN_CONTROLLER/4(DynDef Trigger)
  [GainSetBusy] -> DynamicNoiseFloorAdjustment/5(GainSetBusy)
  [PauseAGC] -> DynamicNoiseFloorAdjustment/9(PauseAGC)
  long_corr_in/1 -> Delay9/1
  [SampleValid] -> SATURATION_DETECTOR/4(RxValid)
  [RxValid] -> MEASURE_AVGPWR/4(RxValid)
  [RxValid] -> DC_REMOVAL/3(RxValid)
  Sample Clock Selection/2(SampleValid) -> [SampleValid]
  PACKET_DETECTION/2(CCA) -> WSD_CCA/1
  [regAGC_MaskWARPPktDet] -> WSD_MASK_WARP_PKT_DET/1
  lte_sync2_in/1 -> Delay10/1
  [GainSetBusy] -> DC_REMOVAL/4(GainSetBusy)
  Convert For WARPLab/1(UFix10_0) -> Delay14/1
  Convert7/1 -> cond_i_out_wl/1
  Convert8/1 -> cond_q_out_wl/1
  raw_i_in/1 -> Delay5/1
  raw_q_in/1 -> Delay13/1
  Delay4/1 -> [GainSetMaster_DONE]
  Delay3/1 -> [CurrentGainSetting]
  Delay2/1 -> [GainSetBusy]
  Delay7/1 -> Convert5/1, Convert9/1
  Delay8/1 -> Convert10/1, Convert6/1
  Delay9/1 -> [cs_longcorrin]
  Delay10/1 -> [LTS_SYNC_2_IN], [cs_lts_sync_2]
  TOP_LEVEL_AGC_TIMING/3(ResetAGC) -> [Reset_FSM]
  TOP_LEVEL_AGC_TIMING/1(FSM_Enable) -> [FSM_Enable]
  Delay6/1 -> Ext_PktDet_Delay/1(Set), [cs_pktdet_in]
  TOP_LEVEL_AGC_TIMING/4(AGC_Done) -> agc_done/1, [AGC_Done]
  [AGC_CurrentState] -> TOP_LEVEL_AGC_TIMING/4(FSM_State)
  [PwrSet_Inc] -> TOP_LEVEL_AGC_TIMING/5(PwrSet_Inc)
  PKT_DET_IN/1 -> Delay6/1
  RESET_AGC/1 -> Logical3/1
  Delay11/1 -> TOP_LEVEL_AGC_TIMING/2(PHY_AGC_Enable)
  Logical3/1 -> Delay12/1
  ENABLE_AGC/1 -> Delay11/1
  TOP_LEVEL_AGC_TIMING/2(Enable_AGC) -> [EnableAGC]
  PAUSE_AGC/1 -> [PauseAGC], Logical3/2
  Delay12/1 -> TOP_LEVEL_AGC_TIMING/3(AGC_Reset)
  Delay1/1 -> DynamicNoiseFloorAdjustment/7(CurrentState)
  Delay5/1 -> [RAW_I]
  Delay13/1 -> [RAW_Q]
  [Reset_FSM] -> Ext_PktDet_Delay/2(Rst)
  Ext_PktDet_Delay/1(Out) -> TOP_LEVEL_AGC_TIMING/1(Pkt_Detect)
  Delay14/1 -> mean_pwr_dbm/1
  DC_REMOVAL/4(Rx_Valid_Out) -> rxvalid_out/1
  Null2/1 -> AGC_GAIN_SELECTION/7(DynDefault_Trigger)
